simulink library "earth_dipole_lib"  (R2016b)
settings: Solver=VariableStepAuto  StartTime=0.0  StopTime=10.0  RelTol=1e-3
undefined symbols (not defined in the file): sim_params
settings Model: Creator=scrice  LastModifiedBy=scrice

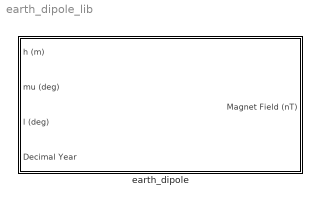
== system earth_dipole_lib ==
  earth_dipole : Subsystem

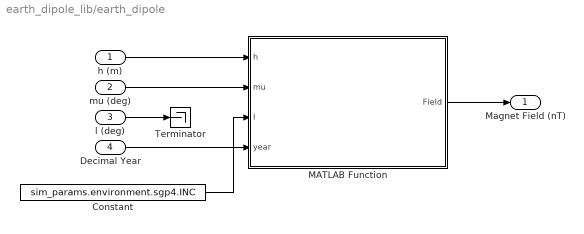
== system earth_dipole_lib/earth_dipole ==
  h (m) : Inport
  mu (deg) : Inport  Port=2
  l (deg) : Inport  Port=3
  Decimal Year : Inport  Port=4
  Constant : Constant  Value=sim_params.environment.sgp4.INC
  MATLAB Function : MATLAB Function  TreatAsAtomicUnit=on
  Terminator : Terminator
  Magnet Field (nT) : Outport
  wires:
  h (m)/1 -> MATLAB Function/1(h)
  mu (deg)/1 -> MATLAB Function/2(mu)
  l (deg)/1 -> Terminator/1
  Decimal Year/1 -> MATLAB Function/4(year)
  MATLAB Function/1(Field) -> Magnet Field (nT)/1
  Constant/1 -> MATLAB Function/3(I)

== matlab function earth_dipole_lib/earth_dipole/MATLAB Function ==
  data: h input; Field output; mu input; I input; year input
function Field = earth_dipole(h,mu,I,year)
    mu_0 = 1.25663706e-6;

    %[XYZ, H, DEC, DIP, F] = wrldmagm(718000, 0, 0, decyear(2015,7,4),'2015')
    %F*1e-8/mu_0
    Heq = 17.28;   %Equitorial field strength found from wgmm
    
    H1 = 3*Heq*sin(I)*cos(I)*sind(mu)^2;
    H2 = -3*Heq*sin(I)*sind(mu)*cosd(mu);
    H3 = Heq*(1-3*sin(I)^2*sind(mu)^2);

Field = mu_0*[H1,H2,H3]';
